simulink model "SWC_APP_type"  (R2024a)
settings: Solver=FixedStepDiscrete  StartTime=0.0  StopTime=10.0  FixedStep=0.001  RelTol=1e-3
values from neighbouring files (symbols this model uses):
  TRUE = boolean( 1 )    [vcu_local_hdr.m]
undefined symbols (not defined in the file or in its folder): KAPP_ADCKL15_enum, KAPP_ADCKL30_enum, KFOC_ADCFlyBackTemp_enum, KFOC_ADCMCUTemp_enum, KFOC_ADCMotorUTemp_enum, KFOC_ADCMotorVTemp_enum, KFOC_ADCMotorWTemp_enum, KFOC_ADCOilTemp_enum, KFOC_ADCSicUTemp_enum, KFOC_ADCSicVTemp_enum, KFOC_ADCSicWTemp_enum, KOPM_FakeKL15_flg
libraries: FVT_lib x19, crm_grc x1, eop_grc x1, halin x1, halout x1, inp x1, llc_grc x1, opm_grc x1, syl_grc x1, dgl_grc x1
(part 2 of 2)

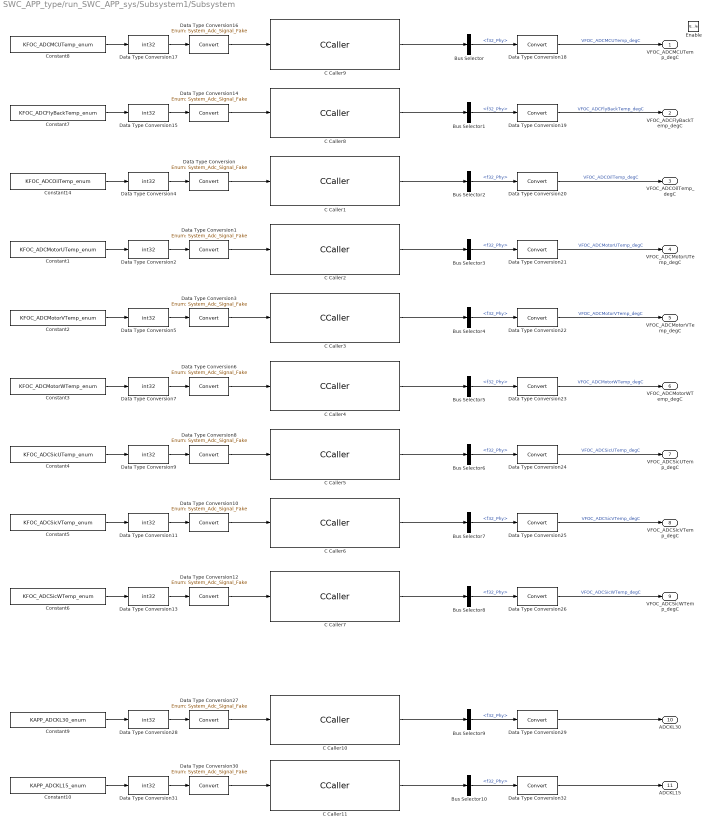
== system SWC_APP_type/run_SWC_APP_sys/Subsystem1/Subsystem ==
  Enable : EnablePort
  Bus Selector{,1..10} (11 alike) : BusSelector  OutputSignals=f32_Phy
  C Caller{1..11} (11 alike) : CCaller  FunctionName=read_adc_system_value  PortSpecificationStruct="%)30     .    ^ ,   8    (     @         %    \"     (    !     0         %  0 \"0    $    _    07)G3F%M90  4&]R=$YA;64 4V-O<&4     26YD97@     5'EP90      4VEZ90      27-';&]B86P   X    P    !@    @    $          4    (     0    ,    !         !   P!O=70 #@   #     &    \"     0         !0    @    !     P    $         $  # &]U=  .    .     8    (    !          %    \"     $    &     0         0    !@   $]U='!U=   #@   #@    &    \"     8         !0    @    !     0    $         \"0    @               X   !0    !@    @    $          4    (     0   !X    !         !     >    0G5S.B!%=D%D8U]3:6=N86Q$871A5'EP95]&86ME   .    ,     8    (    !          %    \"     $    !     0         0  $ ,0    X    P    !@    @    ) @        4    (     0    $    !          (  0      #@   #@    &    \"     0         !0    @    !    !P    $         $     <   !E4VEG;F%L  X    X    !@    @    $          4    (     0    <    !         !     '    95-I9VYA;  .    .     8    (    !          %    \"     $    %     0         0    !0   $EN<'5T    #@   #@    &    \"     8         !0    @    !     0    $         \"0    @               X   !0    !@    @    $          4    (     0   !P    !         !     <    16YU;3H@4WES=&5M7T%D8U]3:6=N86Q?1F%K90     .    ,     8    (    !          %    \"     $    !     0         0  $ ,0    X    P    !@    @    ) @        4    (     0    $    !          (  0"
  Constant1 : Constant  Value=KFOC_ADCMotorUTemp_enum
  Constant10 : Constant  Value=KAPP_ADCKL15_enum
  Constant14 : Constant  Value=KFOC_ADCOilTemp_enum
  Constant2 : Constant  Value=KFOC_ADCMotorVTemp_enum
  Constant3 : Constant  Value=KFOC_ADCMotorWTemp_enum
  Constant4 : Constant  Value=KFOC_ADCSicUTemp_enum
  Constant5 : Constant  Value=KFOC_ADCSicVTemp_enum
  Constant6 : Constant  Value=KFOC_ADCSicWTemp_enum
  Constant7 : Constant  Value=KFOC_ADCFlyBackTemp_enum
  Constant8 : Constant  Value=KFOC_ADCMCUTemp_enum
  Constant9 : Constant  Value=KAPP_ADCKL30_enum
  Data Type Conversion{,1,3,6,8,10,12,14,16,27,30} (11 alike) : DataTypeConversion  OutDataTypeStr=Enum: System_Adc_Signal_Fake  SaturateOnIntegerOverflow=off  RndMeth=Floor
  Data Type Conversion{2,4..5,7,9,11,13,15,17,28,31} (11 alike) : DataTypeConversion  OutDataTypeStr=int32  SaturateOnIntegerOverflow=off  RndMeth=Floor
  Data Type Conversion{18..26,29,32} (11 alike) : DataTypeConversion  SaturateOnIntegerOverflow=off  RndMeth=Floor
  VFOC_ADCMCUTemp_degC : Outport
  VFOC_ADCFlyBackTemp_degC : Outport  Port=2
  VFOC_ADCOilTemp_degC : Outport  Port=3
  VFOC_ADCMotorUTemp_degC : Outport  Port=4
  VFOC_ADCMotorVTemp_degC : Outport  Port=5
  VFOC_ADCMotorWTemp_degC : Outport  Port=6
  VFOC_ADCSicUTemp_degC : Outport  Port=7
  VFOC_ADCSicVTemp_degC : Outport  Port=8
  VFOC_ADCSicWTemp_degC : Outport  Port=9
  ADCKL30 : Outport  Port=10
  ADCKL15 : Outport  Port=11
  wires:
  Data Type Conversion7/1 -> Data Type Conversion6/1
  Constant3/1 -> Data Type Conversion7/1
  C Caller4/1 -> Bus Selector5/1
  Data Type Conversion19/1 -> VFOC_ADCFlyBackTemp_degC/1  "VFOC_ADCFlyBackTemp_degC"
  Data Type Conversion3/1 -> C Caller3/1
  Data Type Conversion23/1 -> VFOC_ADCMotorWTemp_degC/1  "VFOC_ADCMotorWTemp_degC"
  Data Type Conversion/1 -> C Caller1/1
  Constant14/1 -> Data Type Conversion4/1
  Constant5/1 -> Data Type Conversion11/1
  C Caller6/1 -> Bus Selector7/1
  Data Type Conversion14/1 -> C Caller8/1
  Data Type Conversion21/1 -> VFOC_ADCMotorUTemp_degC/1  "VFOC_ADCMotorUTemp_degC"
  C Caller5/1 -> Bus Selector6/1
  Data Type Conversion10/1 -> C Caller6/1
  Data Type Conversion16/1 -> C Caller9/1
  C Caller1/1 -> Bus Selector2/1
  Data Type Conversion12/1 -> C Caller7/1
  Data Type Conversion24/1 -> VFOC_ADCSicUTemp_degC/1  "VFOC_ADCSicUTemp_degC"
  Bus Selector7/1 -> Data Type Conversion25/1  "<f32_Phy>"
  Data Type Conversion8/1 -> C Caller5/1
  Data Type Conversion26/1 -> VFOC_ADCSicWTemp_degC/1  "VFOC_ADCSicWTemp_degC"
  Data Type Conversion9/1 -> Data Type Conversion8/1
  Bus Selector6/1 -> Data Type Conversion24/1  "<f32_Phy>"
  Data Type Conversion17/1 -> Data Type Conversion16/1
  Constant2/1 -> Data Type Conversion5/1
  Bus Selector5/1 -> Data Type Conversion23/1  "<f32_Phy>"
  Constant4/1 -> Data Type Conversion9/1
  C Caller3/1 -> Bus Selector4/1
  Data Type Conversion11/1 -> Data Type Conversion10/1
  C Caller9/1 -> Bus Selector/1
  Constant1/1 -> Data Type Conversion2/1
  C Caller7/1 -> Bus Selector8/1
  Data Type Conversion15/1 -> Data Type Conversion14/1
  Data Type Conversion4/1 -> Data Type Conversion/1
  Bus Selector3/1 -> Data Type Conversion21/1  "<f32_Phy>"
  Data Type Conversion22/1 -> VFOC_ADCMotorVTemp_degC/1  "VFOC_ADCMotorVTemp_degC"
  Constant6/1 -> Data Type Conversion13/1
  Data Type Conversion13/1 -> Data Type Conversion12/1
  C Caller8/1 -> Bus Selector1/1
  Bus Selector2/1 -> Data Type Conversion20/1  "<f32_Phy>"
  C Caller2/1 -> Bus Selector3/1
  Bus Selector1/1 -> Data Type Conversion19/1  "<f32_Phy>"
  Constant7/1 -> Data Type Conversion15/1
  Bus Selector8/1 -> Data Type Conversion26/1  "<f32_Phy>"
  Data Type Conversion2/1 -> Data Type Conversion1/1
  Data Type Conversion6/1 -> C Caller4/1
  Data Type Conversion5/1 -> Data Type Conversion3/1
  Bus Selector/1 -> Data Type Conversion18/1  "<f32_Phy>"
  Data Type Conversion25/1 -> VFOC_ADCSicVTemp_degC/1  "VFOC_ADCSicVTemp_degC"
  Data Type Conversion1/1 -> C Caller2/1
  Constant8/1 -> Data Type Conversion17/1
  Bus Selector4/1 -> Data Type Conversion22/1  "<f32_Phy>"
  Data Type Conversion20/1 -> VFOC_ADCOilTemp_degC/1  "VFOC_ADCOilTemp_degC"
  Data Type Conversion18/1 -> VFOC_ADCMCUTemp_degC/1  "VFOC_ADCMCUTemp_degC"
  Bus Selector9/1 -> Data Type Conversion29/1  "<f32_Phy>"
  Data Type Conversion28/1 -> Data Type Conversion27/1
  Constant9/1 -> Data Type Conversion28/1
  C Caller10/1 -> Bus Selector9/1
  Data Type Conversion27/1 -> C Caller10/1
  Data Type Conversion29/1 -> ADCKL30/1
  Data Type Conversion30/1 -> C Caller11/1
  Constant10/1 -> Data Type Conversion31/1
  C Caller11/1 -> Bus Selector10/1
  Data Type Conversion31/1 -> Data Type Conversion30/1
  Bus Selector10/1 -> Data Type Conversion32/1  "<f32_Phy>"
  Data Type Conversion32/1 -> ADCKL15/1
